simulink subsystem "PropulsionSystem"  (R2024b)
settings: Solver=VariableStepAuto  StartTime=0.0  StopTime=10.0  RelTol=1e-3
model mask{RotorArm=0, Kp=0.05, Ki=0.005, Kd=0, N=100}
  mask prompts: RotorArm "Rotor Arm"
libraries: fl_lib x1
settings Model: Creator=jjha  LastModifiedBy=jjha
settings RTWCC: GPUComputeCapability=3.5

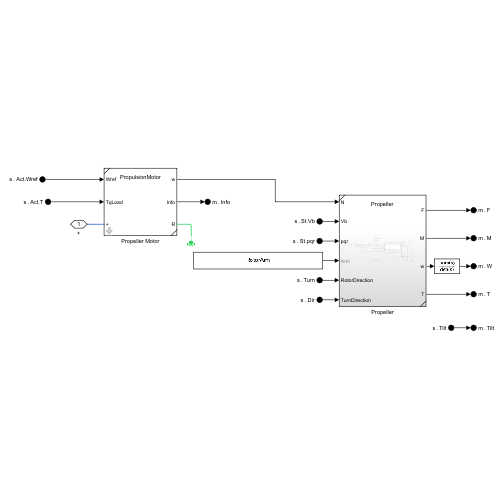
[thumbnail: Simulink's stored preview of the top-level diagram]
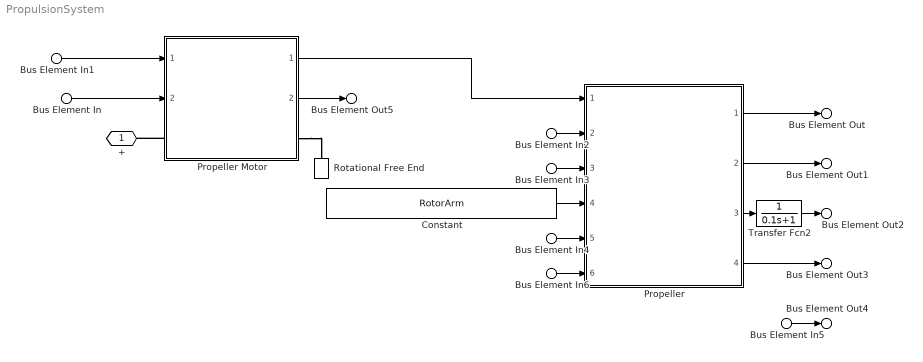
== system PropulsionSystem ==
  Bus Element In4 : Inport  PortName=s  Element=Turn
  Bus Element In5 : Inport  PortName=s  Element=Tilt
  Bus Element In3 : Inport  PortName=s  Element=St.pqr
  Bus Element In2 : Inport  PortName=s  Element=St.Vb
  Bus Element In1 : Inport  PortName=s  Element=Act.Wref
  Bus Element In : Inport  PortName=s  Element=Act.T
  Bus Element In6 : Inport  PortName=s  Element=Dir
  Constant : Constant  Value=RotorArm
  Propeller : Subsystem  ReferencedSubsystem=Propeller
  Propeller Motor : Subsystem  ReferencedSubsystem=PropulsionMotor  Kp=Kp  Ki=Ki  Kd=Kd  N=N
  Rotational Free End : fl_lib/Mechanical/Rotational Elements/Rotational Free End  w_specify=off  w_priority=None  w=0 rad/s  w_nominal_specify=off  w_nominal_value=1  w_nominal_unit=rad/s
  Transfer Fcn2 : TransferFcn  Denominator=[0.1 1]  AbsoluteTolerance=1e-3
  + : PMIOPort  Side=Right
  Bus Element Out : Outport  PortName=m  Element=F
  Bus Element Out1 : Outport  PortName=m  Element=M
  Bus Element Out2 : Outport  PortName=m  Element=W
  Bus Element Out3 : Outport  PortName=m  Element=T
  Bus Element Out4 : Outport  PortName=m  Element=Tilt
  Bus Element Out5 : Outport  PortName=m  Element=Info
  wires:
  Bus Element In4/1 -> Propeller/5
  Constant/1 -> Propeller/4
  Bus Element In6/1 -> Propeller/6
  Bus Element In3/1 -> Propeller/3
  Bus Element In/1 -> Propeller Motor/2
  Propeller/1 -> Bus Element Out/1
  Propeller/2 -> Bus Element Out1/1
  Propeller/3 -> Transfer Fcn2/1
  Propeller/4 -> Bus Element Out3/1
  Transfer Fcn2/1 -> Bus Element Out2/1
  Bus Element In5/1 -> Bus Element Out4/1
  Bus Element In2/1 -> Propeller/2
  Propeller Motor/2 -> Bus Element Out5/1
  Bus Element In1/1 -> Propeller Motor/1
  Propeller Motor/1 -> Propeller/1
  connections:
  Propeller Motor/LConn1 -- +/RConn1
  Propeller Motor/RConn1 -- Rotational Free End/LConn1
